simulink model "primo_simulink"  (R2022b)
settings: Solver=VariableStepAuto  StartTime=0.0  StopTime=10.0  RelTol=1e-3
values from neighbouring files (symbols this model uses):
  den = sym2poly((s+1)^3)    [primosim.m]
  num = sym2poly(10*(1+s*0))    [primosim.m]
settings Model: Creator=danie  LastModifiedBy=danie

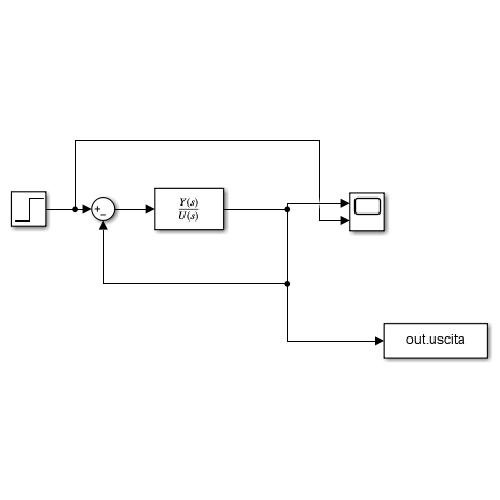
[thumbnail: Simulink's stored preview of the top-level diagram]
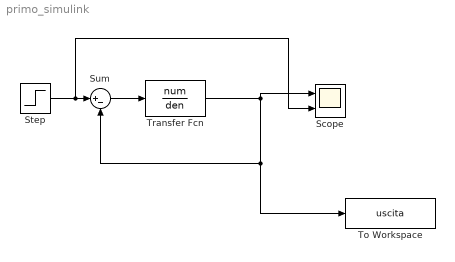
== system primo_simulink ==
  Scope : Scope  NumInputPorts=2
  Step : Step  SampleTime=0
  Sum : Sum  Inputs=|+-
  To Workspace : ToWorkspace  VariableName=uscita  SaveFormat=Timeseries  SampleTime=-1
  Transfer Fcn : TransferFcn  Numerator=num  Denominator=den
  wires:
  Step/1 -> Scope/2, Sum/1
  Transfer Fcn/1 -> Sum/2, To Workspace/1, Scope/1
  Sum/1 -> Transfer Fcn/1
